simulink model "Ejercicio3_espacio_estados"  (R2020a)
settings: Solver=VariableStepAuto  StartTime=0.0  StopTime=60  MaxStep=0.01  RelTol=1e-3
undefined symbols (not defined in the file or in its folder): A, B, C1, C2, D
settings Model: Creator=LENOVO  LastModifiedBy=juan

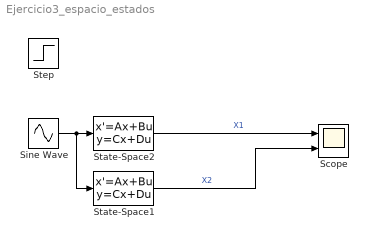
== system Ejercicio3_espacio_estados ==
  Scope : Scope  NumInputPorts=2
  Sine Wave : Sin  SampleTime=0
  State-Space1 : StateSpace  A=A  B=B  C=C2  D=D  InitialCondition=0
  State-Space2 : StateSpace  A=A  B=B  C=C1  D=D  InitialCondition=0
  Step : Step  SampleTime=0
  wires:
  Sine Wave/1 -> State-Space2/1, State-Space1/1
  State-Space1/1 -> Scope/2  "X2"
  State-Space2/1 -> Scope/1  "X1"
